simulink model "three_phase_inverter_dq_control"  (R2022a)
settings: Solver=VariableStepAuto  StartTime=0.0  StopTime=1  RelTol=1e-3
values from neighbouring files (symbols this model uses):
  C_filter = 100e-6    (= 0.0001)    [q1.m]    (also in q2.m; q4.m = 2e-06)
  Ki_current = L_filter*Wn^2    (= 15791.3670417)    [q1.m]    (also in q2.m = 63165.468167; q4.m = 493.480220054)
  Ki_voltage = C_filter*Wn^2    (= 3.55305758439)    [q1.m]    (also in q4.m = 0.0710611516878)
  Kp_current = 2*L_filter*DF*Wn    (= 110.584061406)    [q1.m]    (also in q2.m = 71.0753921948; q4.m = 5.49778714378)
  Kp_voltage = 2*C_filter*DF*Wn    (= 0.0565486677646)    [q1.m]    (also in q4.m = 0.00791681348705)
  L_filter = 40e-3    (= 0.04)    [q1.m]    (also in q2.m; q4.m = 0.00125)
  L_load = sqrt((R_load * V_rms^2)/P_load - R_load^2) / w    [q1.m]    (also in q4.m)
  R_load = (V_rms^2) * (pf_load^2) / P_load    (= 43.32)    [q1.m]    (also in q4.m)
  Tcs = 100*Ts    (= 0.0001)    [q1.m]    (also in q4.m)
libraries: spsabctodq0Lib x5, spsdq0toabcLib x1
settings Model: Creator=fiendchain  LastModifiedBy=acidi

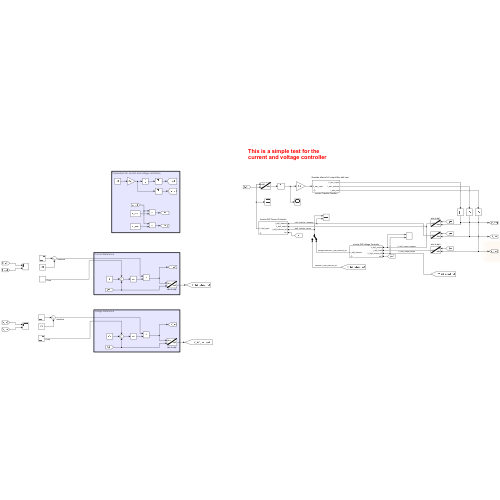
[thumbnail: Simulink's stored preview of the top-level diagram]
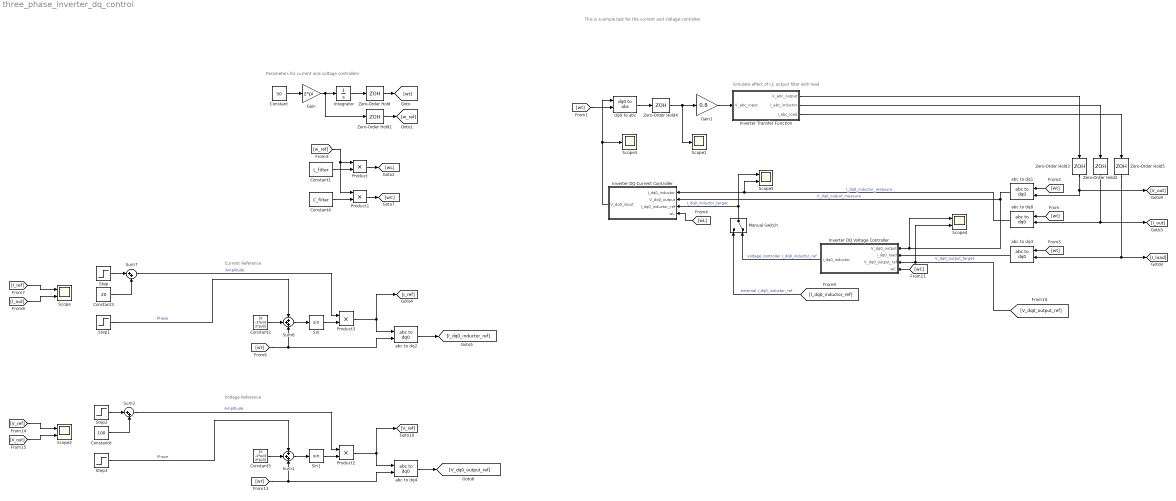
== system three_phase_inverter_dq_control ==
  note: Simulate effect of LC output filter with load
  note: Parameters for current and voltage controllers
  note: This is a simple test for the current and voltage controller
  note: Current Reference
  note: Voltage Reference
  Constant : Constant  Value=50
  Constant1 : Constant  Value=L_filter
  Constant2 : Constant  Value=[0 -2*pi/3 2*pi/3]
  Constant3 : Constant  Value=20
  Constant4 : Constant  Value=C_filter
  Constant5 : Constant  Value=[0 -2*pi/3 2*pi/3]
  Constant6 : Constant  Value=100
  Gain : Gain  Gain=2*pi
  Gain1 : Gain  Gain=0.8
  Integrator : Integrator
  Inverter DQ Current Controller : Subsystem  mask{Kp=Kp_current, Ki=Ki_current}
  Inverter DQ Voltage Controller : Subsystem  mask{Kp=Kp_voltage, Ki=Ki_voltage}
  Inverter Transfer Function : Subsystem  mask{L1=L_filter, C=C_filter, R=R_load, L2=L_load}
      mask prompts: L1 "L_filter"; C "C_filter"; R "R_load"; L2 "L_load"
  Manual Switch : ManualSwitch  CurrentSetting=0
  Product{,1..3} (4 alike) : Product
  Scope{,2,4..5} (4 alike) : Scope  NumInputPorts=2
  Scope1 : Scope
  Scope3 : Scope
  Sin : Trigonometry
  Sin1 : Trigonometry
  Step : Step  Time=0.2  After=4  SampleTime=0
  Step1 : Step  Time=0.4  After=100 * pi/180  SampleTime=0
  Step2 : Step  Time=0.2  After=10  SampleTime=0
  Step3 : Step  Time=0.4  After=100 * pi/180  SampleTime=0
  Sum1 : Sum  Inputs=+++
  Sum2 : Sum  Inputs=|++
  Sum6 : Sum  Inputs=+++
  Sum7 : Sum  Inputs=|++
  Zero-Order Hold{,1..5} (6 alike) : ZeroOrderHold  SampleTime=Tcs
  abc to dq{0..4} (5 alike) : spsabctodq0Lib/abc to dq0  Alignment=Aligned with phase A axis
  dq0 to abc : spsdq0toabcLib/dq0 to abc  Alignment=Aligned with phase A axis
  wires:
  dq0 to abc/1 -> Zero-Order Hold4/1
  [wt] -> abc to dq0/2
  Constant/1 -> Gain/1
  Gain/1 -> Zero-Order Hold1/1, Integrator/1
  Integrator/1 -> Zero-Order Hold/1
  [wt] -> dq0 to abc/2
  [wt] -> abc to dq1/2
  [w_ref] -> Product/1, Product1/1
  Constant1/1 -> Product/2
  Product/1 -> [wL]
  [I_dq0_inductor_ref] -> Manual Switch/1  "external I_dq0_inductor_ref"
  [wt] -> Sum6/3, abc to dq2/2
  Product3/1 -> abc to dq2/1, [I_ref]
  Sin/1 -> Product3/2
  Constant2/1 -> Sum6/2
  Sum6/1 -> Sin/1
  [I_ref] -> Scope/1
  [I_out] -> Scope/2
  Sum7/1 -> Product3/1  "Amplitude"
  Step1/1 -> Sum6/1  "Phase"
  Zero-Order Hold/1 -> [wt]
  Zero-Order Hold1/1 -> [w_ref]
  Zero-Order Hold2/1 -> abc to dq0/1, [I_out]
  Zero-Order Hold3/1 -> [V_out], abc to dq1/1
  Zero-Order Hold4/1 -> Scope1/1, Gain1/1
  Step/1 -> Sum7/1
  Constant3/1 -> Sum7/2
  [wL] -> Inverter DQ Current Controller/4(wL)
  Inverter Transfer Function/1(V_abc_output) -> Zero-Order Hold3/1
  Inverter Transfer Function/2(I_abc_inductor) -> Zero-Order Hold2/1
  Inverter DQ Current Controller/1(V_dq0_input) -> dq0 to abc/1, Scope3/1
  Inverter Transfer Function/3(I_abc_load) -> Zero-Order Hold5/1
  [wt] -> abc to dq3/2
  Zero-Order Hold5/1 -> [I_load], abc to dq3/1
  abc to dq3/1 -> Inverter DQ Voltage Controller/2(i_dq0_load)
  Constant4/1 -> Product1/2
  Product1/1 -> [wC]
  [wC] -> Inverter DQ Voltage Controller/4(wC)
  Manual Switch/1 -> Inverter DQ Current Controller/3(I_dq0_inductor_ref), Scope5/1  "I_dq0_inductor_target"
  Inverter DQ Voltage Controller/1(i_dq0_inductor) -> Manual Switch/2  "voltage controller I_dq0_inductor_ref"
  abc to dq1/1 -> Inverter DQ Current Controller/2(V_dq0_output), Scope4/1, Inverter DQ Voltage Controller/1(V_dq0_output)  "V_dq0_output_measure"
  abc to dq0/1 -> Inverter DQ Current Controller/1(I_dq0_inductor), Scope5/2  "I_dq0_inductor_measure"
  Sum1/1 -> Sin1/1
  [wt] -> Sum1/3, abc to dq4/2
  Constant6/1 -> Sum2/2
  Step3/1 -> Sum1/1  "Phase"
  Constant5/1 -> Sum1/2
  [V_ref] -> Scope2/1
  Sin1/1 -> Product2/2
  Sum2/1 -> Product2/1  "Ampltiude"
  Product2/1 -> abc to dq4/1, [V_ref]
  Step2/1 -> Sum2/1
  [V_out] -> Scope2/2
  [V_dq0_output_ref] -> Scope4/2, Inverter DQ Voltage Controller/3(V_dq0_output_ref)  "V_dq0_output_target"
  Gain1/1 -> Inverter Transfer Function/1(V_abc_input)
  abc to dq2/1 -> [I_dq0_inductor_ref]
  abc to dq4/1 -> [V_dq0_output_ref]

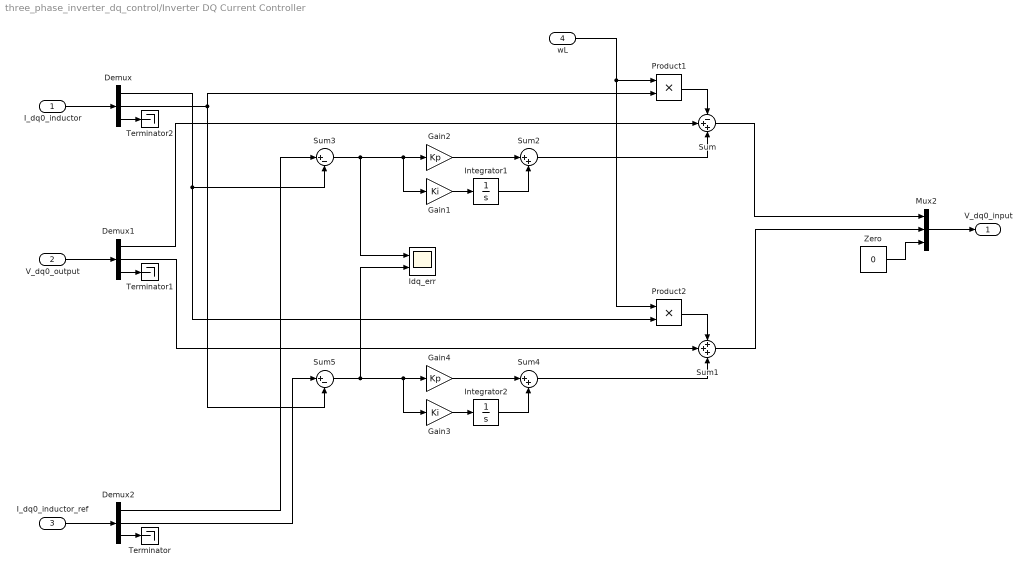
== system three_phase_inverter_dq_control/Inverter DQ Current Controller ==
  I_dq0_inductor : Inport
  V_dq0_output : Inport  Port=2
  I_dq0_inductor_ref : Inport  Port=3
  wL : Inport  Port=4
  Demux : Demux  Outputs=3
  Demux1 : Demux  Outputs=3
  Demux2 : Demux  Outputs=3
  Gain1 : Gain  Gain=Ki
  Gain2 : Gain  Gain=Kp
  Gain3 : Gain  Gain=Ki
  Gain4 : Gain  Gain=Kp
  Idq_err : Scope  NumInputPorts=2
  Integrator1 : Integrator  UpperSaturationLimit=10000  LowerSaturationLimit=-10000
  Integrator2 : Integrator
  Mux2 : Mux  Inputs=3
  Product1 : Product
  Product2 : Product
  Sum : Sum  Inputs=-++
  Sum1 : Sum  Inputs=+++
  Sum2 : Sum  Inputs=|++
  Sum3 : Sum  Inputs=|+-
  Sum4 : Sum  Inputs=|++
  Sum5 : Sum  Inputs=|+-
  Terminator : Terminator
  Terminator1 : Terminator
  Terminator2 : Terminator
  Zero : Constant  Value=0  OutDataTypeStr=Inherit: Inherit via back propagation
  V_dq0_input : Outport
  wires:
  Gain3/1 -> Integrator2/1
  I_dq0_inductor_ref/1 -> Demux2/1
  V_dq0_output/1 -> Demux1/1
  Demux2/1 -> Sum3/1
  Integrator1/1 -> Sum2/2
  Gain4/1 -> Sum4/1
  Product2/1 -> Sum1/1
  Sum5/1 -> Idq_err/2, Gain4/1, Gain3/1
  Mux2/1 -> V_dq0_input/1
  Demux/2 -> Sum5/2, Product1/2
  Demux/1 -> Sum3/2, Product2/2
  Sum3/1 -> Idq_err/1, Gain2/1, Gain1/1
  Demux2/3 -> Terminator/1
  I_dq0_inductor/1 -> Demux/1
  Sum/1 -> Mux2/1
  Demux1/1 -> Sum/2
  Integrator2/1 -> Sum4/2
  Product1/1 -> Sum/1
  Gain2/1 -> Sum2/1
  Sum2/1 -> Sum/3
  Gain1/1 -> Integrator1/1
  Sum1/1 -> Mux2/2
  Zero/1 -> Mux2/3
  Sum4/1 -> Sum1/3
  Demux1/2 -> Sum1/2
  Demux2/2 -> Sum5/1
  Demux1/3 -> Terminator1/1
  Demux/3 -> Terminator2/1
  wL/1 -> Product2/1, Product1/1

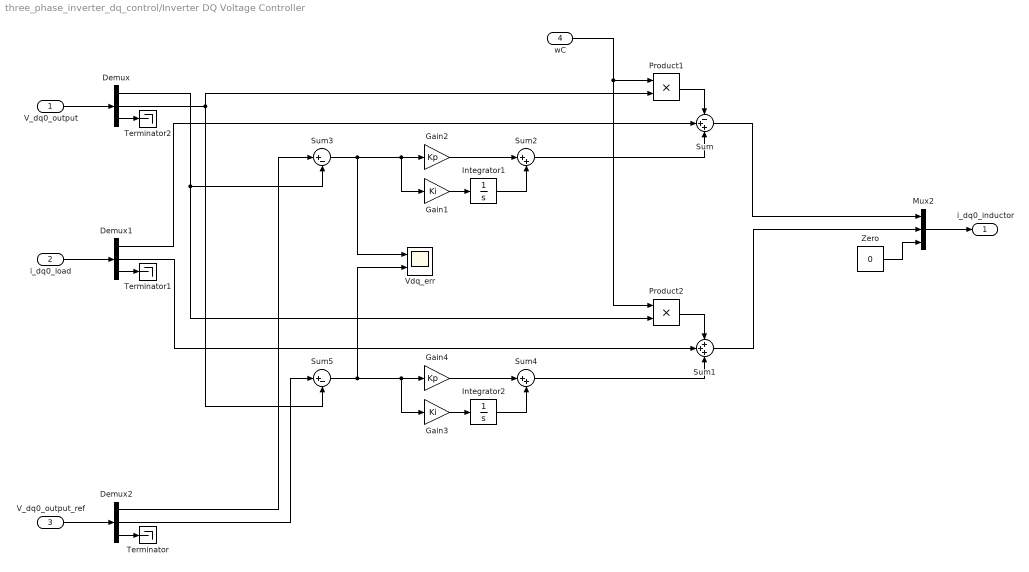
== system three_phase_inverter_dq_control/Inverter DQ Voltage Controller ==
  V_dq0_output : Inport
  i_dq0_load : Inport  Port=2
  V_dq0_output_ref : Inport  Port=3
  wC : Inport  Port=4
  Demux : Demux  Outputs=3
  Demux1 : Demux  Outputs=3
  Demux2 : Demux  Outputs=3
  Gain1 : Gain  Gain=Ki
  Gain2 : Gain  Gain=Kp
  Gain3 : Gain  Gain=Ki
  Gain4 : Gain  Gain=Kp
  Integrator1 : Integrator  UpperSaturationLimit=10000  LowerSaturationLimit=-10000
  Integrator2 : Integrator
  Mux2 : Mux  Inputs=3
  Product1 : Product
  Product2 : Product
  Sum : Sum  Inputs=-++
  Sum1 : Sum  Inputs=+++
  Sum2 : Sum  Inputs=|++
  Sum3 : Sum  Inputs=|+-
  Sum4 : Sum  Inputs=|++
  Sum5 : Sum  Inputs=|+-
  Terminator : Terminator
  Terminator1 : Terminator
  Terminator2 : Terminator
  Vdq_err : Scope  NumInputPorts=2
  Zero : Constant  Value=0  OutDataTypeStr=Inherit: Inherit via back propagation
  i_dq0_inductor : Outport
  wires:
  Gain3/1 -> Integrator2/1
  V_dq0_output_ref/1 -> Demux2/1
  i_dq0_load/1 -> Demux1/1
  Demux2/1 -> Sum3/1
  Integrator1/1 -> Sum2/2
  Gain4/1 -> Sum4/1
  Product2/1 -> Sum1/1
  Sum5/1 -> Vdq_err/2, Gain4/1, Gain3/1
  Mux2/1 -> i_dq0_inductor/1
  Demux/2 -> Sum5/2, Product1/2
  Demux/1 -> Sum3/2, Product2/2
  Sum3/1 -> Vdq_err/1, Gain2/1, Gain1/1
  Demux2/3 -> Terminator/1
  V_dq0_output/1 -> Demux/1
  Sum/1 -> Mux2/1
  Demux1/1 -> Sum/2
  Integrator2/1 -> Sum4/2
  Product1/1 -> Sum/1
  Gain2/1 -> Sum2/1
  Sum2/1 -> Sum/3
  Gain1/1 -> Integrator1/1
  Sum1/1 -> Mux2/2
  Zero/1 -> Mux2/3
  Sum4/1 -> Sum1/3
  Demux1/2 -> Sum1/2
  Demux2/2 -> Sum5/1
  Demux1/3 -> Terminator1/1
  Demux/3 -> Terminator2/1
  wC/1 -> Product2/1, Product1/1

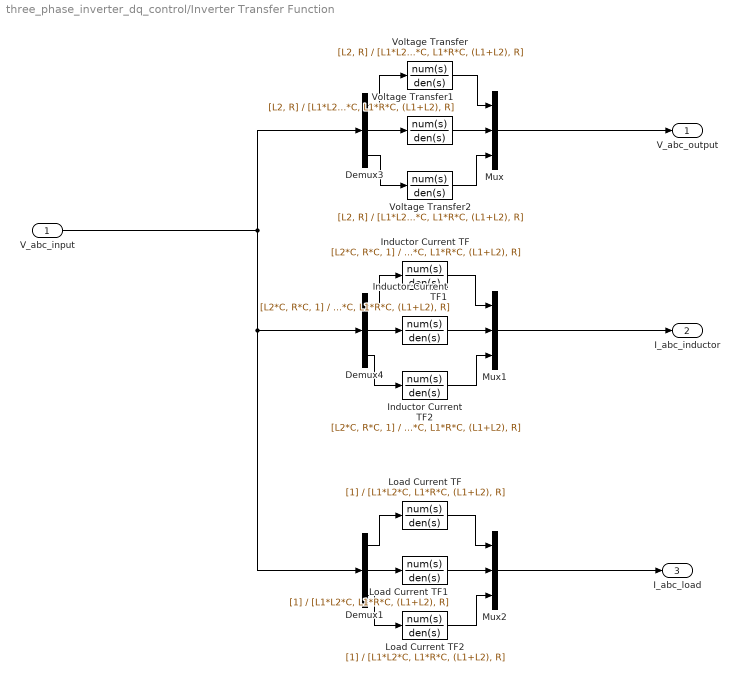
== system three_phase_inverter_dq_control/Inverter Transfer Function ==
  V_abc_input : Inport
  Demux1 : Demux  Outputs=3
  Demux3 : Demux  Outputs=3
  Demux4 : Demux  Outputs=3
  Inductor Current TF : TransferFcn  Numerator=[L2*C, R*C, 1]  Denominator=[L1*L2*C, L1*R*C, (L1+L2), R]
  Inductor Current TF1 : TransferFcn  Numerator=[L2*C, R*C, 1]  Denominator=[L1*L2*C, L1*R*C, (L1+L2), R]
  Inductor Current TF2 : TransferFcn  Numerator=[L2*C, R*C, 1]  Denominator=[L1*L2*C, L1*R*C, (L1+L2), R]
  Load Current TF : TransferFcn  Denominator=[L1*L2*C, L1*R*C, (L1+L2), R]
  Load Current TF1 : TransferFcn  Denominator=[L1*L2*C, L1*R*C, (L1+L2), R]
  Load Current TF2 : TransferFcn  Denominator=[L1*L2*C, L1*R*C, (L1+L2), R]
  Mux : Mux  Inputs=3
  Mux1 : Mux  Inputs=3
  Mux2 : Mux  Inputs=3
  Voltage Transfer : TransferFcn  Numerator=[L2, R]  Denominator=[L1*L2*C, L1*R*C, (L1+L2), R]
  Voltage Transfer1 : TransferFcn  Numerator=[L2, R]  Denominator=[L1*L2*C, L1*R*C, (L1+L2), R]
  Voltage Transfer2 : TransferFcn  Numerator=[L2, R]  Denominator=[L1*L2*C, L1*R*C, (L1+L2), R]
  V_abc_output : Outport
  I_abc_inductor : Outport  Port=2
  I_abc_load : Outport  Port=3
  wires:
  Voltage Transfer2/1 -> Mux/3
  Demux3/2 -> Voltage Transfer1/1
  Inductor Current TF/1 -> Mux1/1
  Demux3/1 -> Voltage Transfer/1
  Demux4/3 -> Inductor Current TF2/1
  Inductor Current TF2/1 -> Mux1/3
  Demux3/3 -> Voltage Transfer2/1
  Demux4/2 -> Inductor Current TF1/1
  Demux4/1 -> Inductor Current TF/1
  Inductor Current TF1/1 -> Mux1/2
  Voltage Transfer/1 -> Mux/1
  Voltage Transfer1/1 -> Mux/2
  Mux/1 -> V_abc_output/1
  V_abc_input/1 -> Demux1/1, Demux4/1, Demux3/1
  Demux1/3 -> Load Current TF2/1
  Load Current TF/1 -> Mux2/1
  Demux1/1 -> Load Current TF/1
  Load Current TF2/1 -> Mux2/3
  Load Current TF1/1 -> Mux2/2
  Demux1/2 -> Load Current TF1/1
  Mux1/1 -> I_abc_inductor/1
  Mux2/1 -> I_abc_load/1
